simulink subsystem "FBRController"  (R2021a)
settings: Solver=VariableStepAuto  StartTime=0.0  StopTime=10.0  RelTol=1e-3
libraries: vrlib x5
settings Model: Creator=chiar  LastModifiedBy=chiar

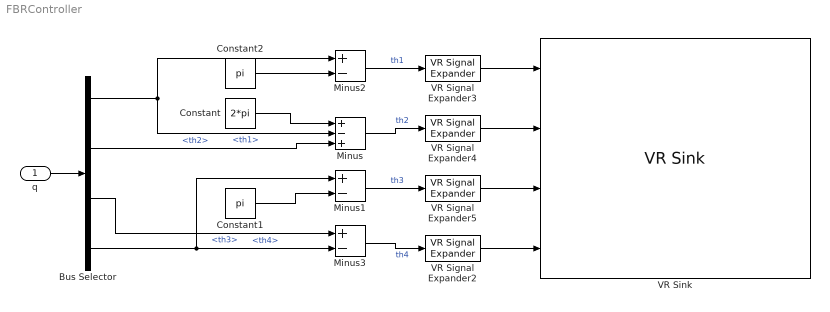
== system FBRController ==
  q : Inport
  Bus Selector : BusSelector  OutputSignals=th1,th2,th3,th4
  Constant : Constant  Value=2*pi
  Constant1 : Constant  Value=pi
  Constant2 : Constant  Value=pi
  Minus : Sum  Inputs=+-+
  Minus1 : Sum  Inputs=+-
  Minus2 : Sum  Inputs=+-
  Minus3 : Sum  Inputs=+-
  VR Signal Expander{2..5} (4 alike) : vrlib/VR Signal Expander  outwidth=4  outidx=4
  VR Sink : vrlib/VR Sink  InstantiateOnLoad=on  SampleTime=0.1  ViewEnable=on  RemoteChange=off  RemoteView=off  FieldsWritten=Link_LA.rotation.4.1.1.double#Link_LB.rotation.4.1.1.double#Link_RA.rotation.4.1.1.double#Link_RB.rotation.4.1.1.double  WorldFileName=FBR3d.x3d  WorldDescription=FiveBarRobot  AutoView=off  VideoDimensions=[]  AllowVariableSize=off
  wires:
  Minus/1 -> VR Signal Expander4/1  "th2"
  Minus1/1 -> VR Signal Expander5/1  "th3"
  Constant/1 -> Minus/1
  Constant2/1 -> Minus2/2
  Minus2/1 -> VR Signal Expander3/1  "th1"
  Minus3/1 -> VR Signal Expander2/1  "th4"
  q/1 -> Bus Selector/1
  Bus Selector/1 -> Minus2/1, Minus/2  "<th1>"
  Bus Selector/4 -> Minus3/2, Minus1/1  "<th4>"
  Bus Selector/2 -> Minus/3  "<th2>"
  Bus Selector/3 -> Minus3/1  "<th3>"
  Constant1/1 -> Minus1/2
  VR Signal Expander3/1 -> VR Sink/1
  VR Signal Expander4/1 -> VR Sink/2
  VR Signal Expander2/1 -> VR Sink/4
  VR Signal Expander5/1 -> VR Sink/3
